simulink model "urineanalylsis"  (R2022a)
settings: Solver=VariableStepAuto  StartTime=0.0  StopTime=10.0  RelTol=1e-3
libraries: simulink x43, simulink_extras x1
settings Model: Creator=user  LastModifiedBy=hp

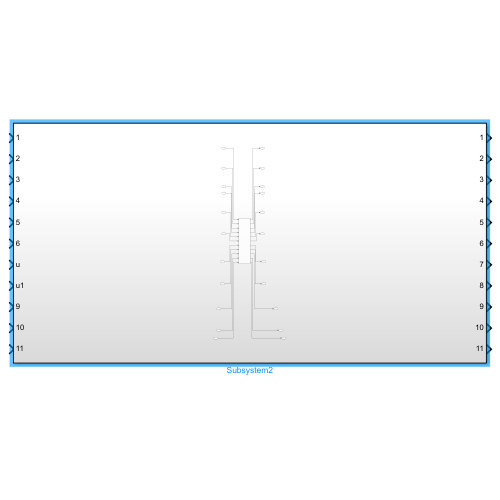
[thumbnail: Simulink's stored preview of the top-level diagram]
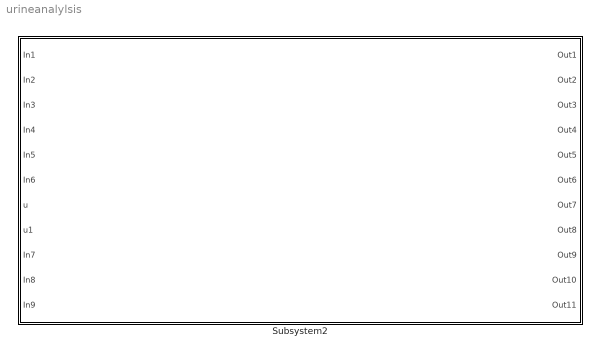
== system urineanalylsis ==
  Subsystem2 : Subsystem

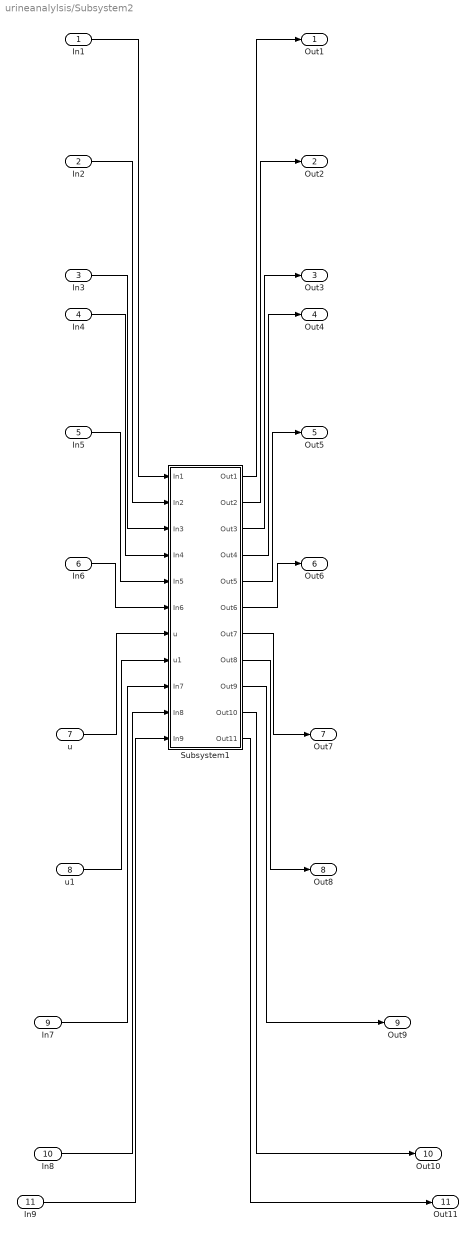
== system urineanalylsis/Subsystem2 ==
  In1 : Inport
  In2 : Inport  Port=2
  In3 : Inport  Port=3
  In4 : Inport  Port=4
  In5 : Inport  Port=5
  In6 : Inport  Port=6
  u : Inport  Port=7
  u1 : Inport  Port=8
  In7 : Inport  Port=9
  In8 : Inport  Port=10
  In9 : Inport  Port=11
  Subsystem1 : Subsystem
  Out1 : Outport
  Out2 : Outport  Port=2
  Out3 : Outport  Port=3
  Out4 : Outport  Port=4
  Out5 : Outport  Port=5
  Out6 : Outport  Port=6
  Out7 : Outport  Port=7
  Out8 : Outport  Port=8
  Out9 : Outport  Port=9
  Out10 : Outport  Port=10
  Out11 : Outport  Port=11
  wires:
  In1/1 -> Subsystem1/1(In1)
  In2/1 -> Subsystem1/2(In2)
  In3/1 -> Subsystem1/3(In3)
  In4/1 -> Subsystem1/4(In4)
  In5/1 -> Subsystem1/5(In5)
  In6/1 -> Subsystem1/6(In6)
  u/1 -> Subsystem1/7(u)
  u1/1 -> Subsystem1/8(u1)
  In7/1 -> Subsystem1/9(In7)
  In8/1 -> Subsystem1/10(In8)
  In9/1 -> Subsystem1/11(In9)
  Subsystem1/1(Out1) -> Out1/1
  Subsystem1/2(Out2) -> Out2/1
  Subsystem1/3(Out3) -> Out3/1
  Subsystem1/4(Out4) -> Out4/1
  Subsystem1/5(Out5) -> Out5/1
  Subsystem1/6(Out6) -> Out6/1
  Subsystem1/7(Out7) -> Out7/1
  Subsystem1/8(Out8) -> Out8/1
  Subsystem1/9(Out9) -> Out9/1
  Subsystem1/10(Out10) -> Out10/1
  Subsystem1/11(Out11) -> Out11/1

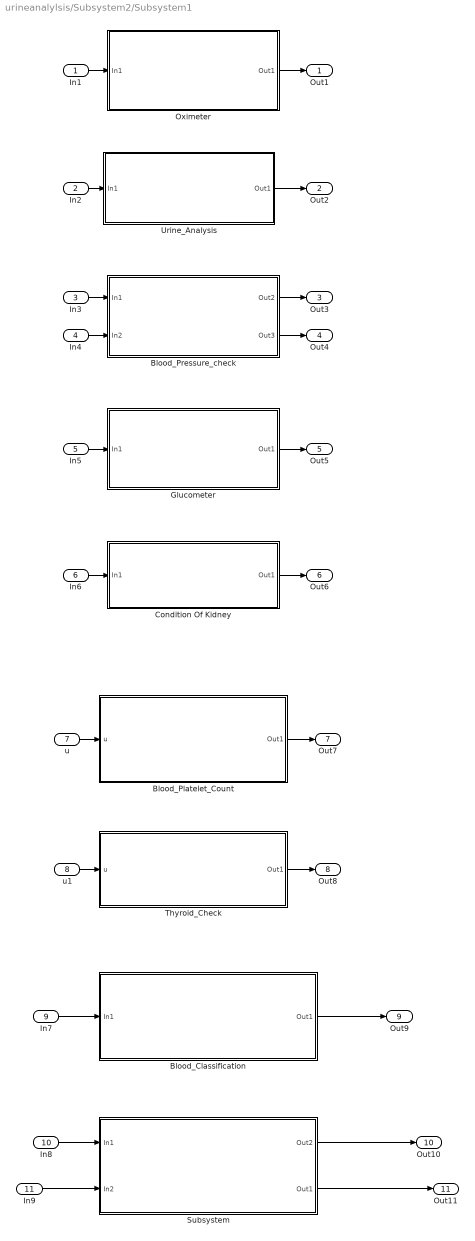
== system urineanalylsis/Subsystem2/Subsystem1 ==
  In1 : Inport
  In2 : Inport  Port=2
  In3 : Inport  Port=3
  In4 : Inport  Port=4
  In5 : Inport  Port=5
  In6 : Inport  Port=6
  u : Inport  Port=7
  u1 : Inport  Port=8
  In7 : Inport  Port=9
  In8 : Inport  Port=10
  In9 : Inport  Port=11
  Blood_Classification : Subsystem
  Blood_Platelet_Count : Subsystem
  Blood_Pressure_check : Subsystem
  Condition Of Kidney : Subsystem
  Glucometer : Subsystem
  Oximeter : Subsystem
  Subsystem : Subsystem
  Thyroid_Check : Subsystem
  Urine_Analysis : Subsystem
  Out1 : Outport
  Out2 : Outport  Port=2
  Out3 : Outport  Port=3
  Out4 : Outport  Port=4
  Out5 : Outport  Port=5
  Out6 : Outport  Port=6
  Out7 : Outport  Port=7
  Out8 : Outport  Port=8
  Out9 : Outport  Port=9
  Out10 : Outport  Port=10
  Out11 : Outport  Port=11
  wires:
  In6/1 -> Condition Of Kidney/1(In1)
  Subsystem/1(Out2) -> Out10/1
  In8/1 -> Subsystem/1(In1)
  In3/1 -> Blood_Pressure_check/1(In1)
  In4/1 -> Blood_Pressure_check/2(In2)
  In7/1 -> Blood_Classification/1(In1)
  u1/1 -> Thyroid_Check/1(u)
  In1/1 -> Oximeter/1(In1)
  u/1 -> Blood_Platelet_Count/1(u)
  Urine_Analysis/1(Out1) -> Out2/1
  Blood_Pressure_check/1(Out2) -> Out3/1
  Blood_Pressure_check/2(Out3) -> Out4/1
  Oximeter/1(Out1) -> Out1/1
  In2/1 -> Urine_Analysis/1(In1)
  Subsystem/2(Out1) -> Out11/1
  Thyroid_Check/1(Out1) -> Out8/1
  Condition Of Kidney/1(Out1) -> Out6/1
  Blood_Classification/1(Out1) -> Out9/1
  Blood_Platelet_Count/1(Out1) -> Out7/1
  In5/1 -> Glucometer/1(In1)
  Glucometer/1(Out1) -> Out5/1
  In9/1 -> Subsystem/2(In2)

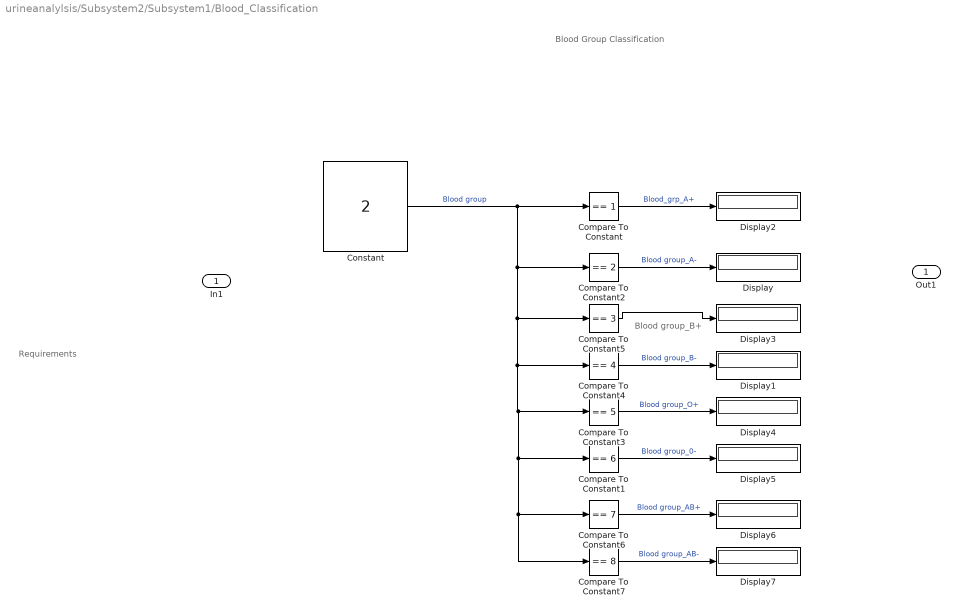
== system urineanalylsis/Subsystem2/Subsystem1/Blood_Classification ==
  note: Requirements
  note: Blood group_B+
  note: Blood Group Classification
  In1 : Inport
  Compare To Constant : simulink/Logic and Bit Operations/Compare To Constant  relop===  const=1  OutDataTypeStr=boolean
  Compare To Constant1 : simulink/Logic and Bit Operations/Compare To Constant  relop===  const=6  OutDataTypeStr=boolean
  Compare To Constant2 : simulink/Logic and Bit Operations/Compare To Constant  relop===  const=2  OutDataTypeStr=boolean
  Compare To Constant3 : simulink/Logic and Bit Operations/Compare To Constant  relop===  const=5  OutDataTypeStr=boolean
  Compare To Constant4 : simulink/Logic and Bit Operations/Compare To Constant  relop===  const=4  OutDataTypeStr=boolean
  Compare To Constant5 : simulink/Logic and Bit Operations/Compare To Constant  relop===  const=3  OutDataTypeStr=boolean
  Compare To Constant6 : simulink/Logic and Bit Operations/Compare To Constant  relop===  const=7  OutDataTypeStr=boolean
  Compare To Constant7 : simulink/Logic and Bit Operations/Compare To Constant  relop===  const=8  OutDataTypeStr=boolean
  Constant : Constant  Value=2
  Display{,1..7} (8 alike) : Display
  Out1 : Outport
  wires:
  Compare To Constant5/1 -> Display3/1
  Compare To Constant4/1 -> Display1/1  "Blood group_B-"
  Constant/1 -> Compare To Constant7/1, Compare To Constant6/1, Compare To Constant1/1, Compare To Constant3/1, Compare To Constant4/1, Compare To Constant5/1, Compare To Constant2/1, Compare To Constant/1  "Blood group"
  Compare To Constant6/1 -> Display6/1  "Blood group_AB+"
  Compare To Constant1/1 -> Display5/1  "Blood group_0-"
  Compare To Constant/1 -> Display2/1  "Blood_grp_A+"
  Compare To Constant2/1 -> Display/1  "Blood group_A-"
  Compare To Constant3/1 -> Display4/1  "Blood group_O+"
  Compare To Constant7/1 -> Display7/1  "Blood group_AB-"

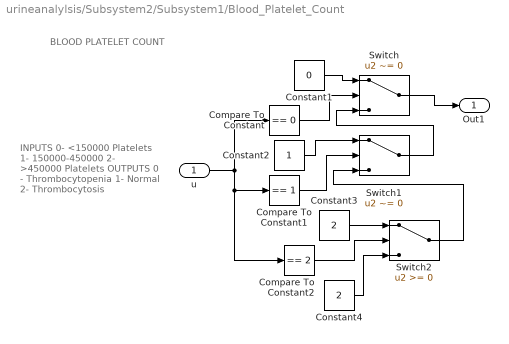
== system urineanalylsis/Subsystem2/Subsystem1/Blood_Platelet_Count ==
  note: BLOOD PLATELET COUNT
  note: INPUTS
      |
      | 0- <150000 Platelets
      | 1- 150000-450000
      | 2- >450000 Platelets
      |
      | OUTPUTS
      | 0 - Thrombocytopenia
      | 1-  Normal
      | 2-  Thrombocytosis
  u : Inport
  Compare To Constant : simulink/Logic and Bit Operations/Compare To Constant  relop===  const=0  OutDataTypeStr=boolean
  Compare To Constant1 : simulink/Logic and Bit Operations/Compare To Constant  relop===  const=1  OutDataTypeStr=boolean
  Compare To Constant2 : simulink/Logic and Bit Operations/Compare To Constant  relop===  const=2  OutDataTypeStr=boolean
  Constant1 : Constant  Value=0
  Constant2 : Constant
  Constant3 : Constant  Value=2
  Constant4 : Constant  Value=2
  Switch : Switch  Criteria=u2 ~= 0  SaturateOnIntegerOverflow=off  InputSameDT=off
  Switch1 : Switch  Criteria=u2 ~= 0  SaturateOnIntegerOverflow=off  InputSameDT=off
  Switch2 : Switch  SaturateOnIntegerOverflow=off  InputSameDT=off
  Out1 : Outport
  wires:
  Switch/1 -> Out1/1
  Constant2/1 -> Switch1/1
  Constant4/1 -> Switch2/3
  Compare To Constant/1 -> Switch/2
  Constant1/1 -> Switch/1
  Compare To Constant2/1 -> Switch2/2
  Compare To Constant1/1 -> Switch1/2
  Switch2/1 -> Switch1/3
  Constant3/1 -> Switch2/1
  Switch1/1 -> Switch/3
  u/1 -> Compare To Constant2/1, Compare To Constant1/1, Compare To Constant/1

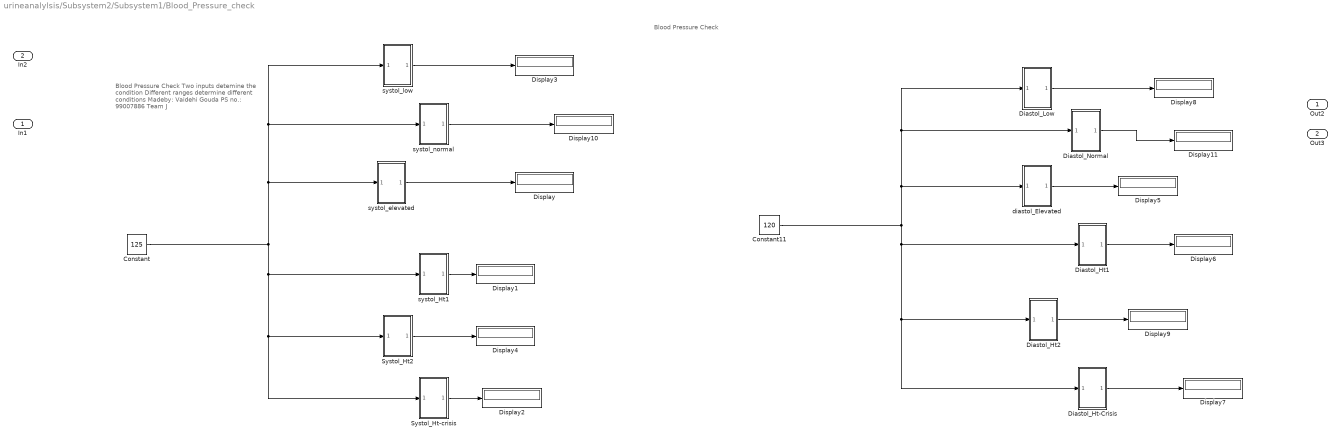
== system urineanalylsis/Subsystem2/Subsystem1/Blood_Pressure_check ==
  note: Blood Pressure Check
      |
      | Two inputs detemine the condition
      | Different ranges determine different conditions
      |
      | Madeby: Vaidehi Gouda
      | PS no.: 99007886
      | Team J
  note: Blood Pressure Check
  In1 : Inport
  In2 : Inport  Port=2
  Constant : Constant  Value=125
  Constant11 : Constant  Value=120
  Diastol_Ht-Crisis : Subsystem
  Diastol_Ht1 : Subsystem
  Diastol_Ht2 : Subsystem
  Diastol_Low : Subsystem
  Diastol_Normal : Subsystem
  Display{,1..11} (12 alike) : Display
  Systol_Ht-crisis : Subsystem
  Systol_Ht2 : Subsystem
  diastol_Elevated : Subsystem
  systol_Ht1 : Subsystem
  systol_elevated : Subsystem
  systol_low : Subsystem
  systol_normal : Subsystem
  Out2 : Outport
  Out3 : Outport  Port=2
  wires:
  Diastol_Ht2/1(Out1) -> Display9/1
  systol_Ht1/1(Out1) -> Display1/1
  Constant/1 -> Systol_Ht-crisis/1(In1), Systol_Ht2/1(In1), systol_Ht1/1(In1), systol_low/1(In1), systol_normal/1(In1), systol_elevated/1(In1)
  Diastol_Ht-Crisis/1(Out1) -> Display7/1
  Systol_Ht2/1(Out1) -> Display4/1
  Diastol_Normal/1(Out1) -> Display11/1
  systol_normal/1(Out1) -> Display10/1
  Constant11/1 -> Diastol_Ht-Crisis/1(In1), Diastol_Ht2/1(In1), Diastol_Ht1/1(In1), Diastol_Low/1(In1), Diastol_Normal/1(In1), diastol_Elevated/1(In1)
  diastol_Elevated/1(Out1) -> Display5/1
  Diastol_Low/1(Out1) -> Display8/1
  Diastol_Ht1/1(Out1) -> Display6/1
  systol_low/1(Out1) -> Display3/1
  Systol_Ht-crisis/1(Out1) -> Display2/1
  systol_elevated/1(Out1) -> Display/1

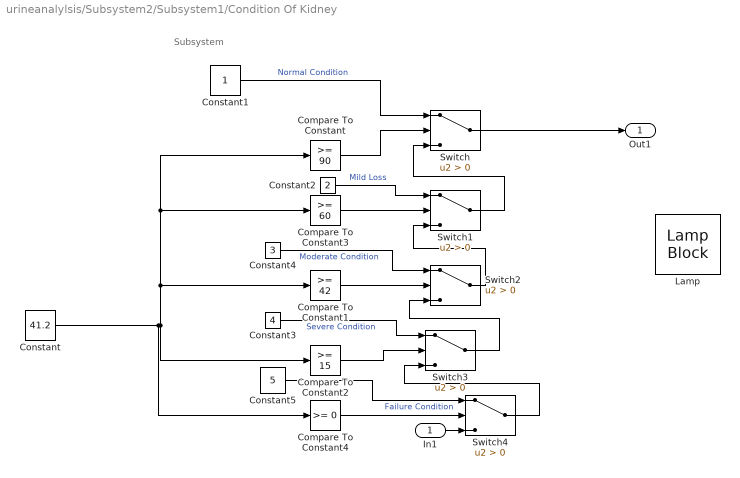
== system urineanalylsis/Subsystem2/Subsystem1/Condition Of Kidney ==
  note: Subsystem
  In1 : Inport
  Compare To Constant : simulink/Logic and Bit Operations/Compare To Constant  relop=>=  const=90  OutDataTypeStr=boolean
  Compare To Constant1 : simulink/Logic and Bit Operations/Compare To Constant  relop=>=  const=42  OutDataTypeStr=boolean
  Compare To Constant2 : simulink/Logic and Bit Operations/Compare To Constant  relop=>=  const=15  OutDataTypeStr=boolean
  Compare To Constant3 : simulink/Logic and Bit Operations/Compare To Constant  relop=>=  const=60  OutDataTypeStr=boolean
  Compare To Constant4 : simulink/Logic and Bit Operations/Compare To Constant  relop=>=  const=0  OutDataTypeStr=boolean
  Constant : Constant  Value=41.2
  Constant1 : Constant
  Constant2 : Constant  Value=2
  Constant3 : Constant  Value=4
  Constant4 : Constant  Value=3
  Constant5 : Constant  Value=5
  Lamp : LampBlock  LabelPosition=Hide
  Switch{,1..4} (5 alike) : Switch  Criteria=u2 > Threshold  SaturateOnIntegerOverflow=off  InputSameDT=off
  Out1 : Outport
  wires:
  Compare To Constant/1 -> Switch/2
  Constant1/1 -> Switch/1  "Normal Condition"
  Compare To Constant4/1 -> Switch4/2
  Switch2/1 -> Switch1/3
  Constant/1 -> Compare To Constant3/1, Compare To Constant/1, Compare To Constant1/1, Compare To Constant2/1, Compare To Constant4/1
  Switch4/1 -> Switch3/3
  Switch1/1 -> Switch/3
  Compare To Constant1/1 -> Switch2/2
  Switch3/1 -> Switch2/3
  Constant3/1 -> Switch3/1  "Severe Condition"
  Constant4/1 -> Switch2/1  "Moderate Condition"
  Compare To Constant2/1 -> Switch3/2
  Compare To Constant3/1 -> Switch1/2
  Constant2/1 -> Switch1/1  "Mild Loss"
  Constant5/1 -> Switch4/1  "Failure Condition"
  In1/1 -> Switch4/3
  Switch/1 -> Out1/1

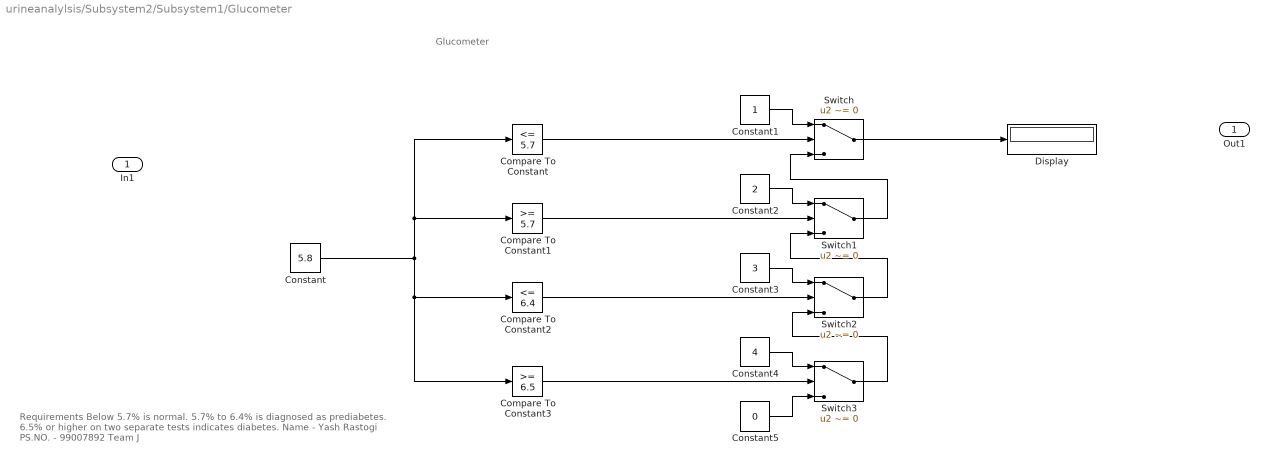
== system urineanalylsis/Subsystem2/Subsystem1/Glucometer ==
  note: Glucometer
  note: Requirements
      |
      | Below 5.7% is normal.
      | 5.7% to 6.4% is diagnosed as prediabetes.
      | 6.5% or higher on two separate tests indicates diabetes.
      | Name - Yash Rastogi
      | PS.NO. - 99007892
      | Team J
  In1 : Inport
  Compare To Constant : simulink/Logic and Bit Operations/Compare To Constant  relop=<=  const=5.7  OutDataTypeStr=boolean
  Compare To Constant1 : simulink/Logic and Bit Operations/Compare To Constant  relop=>=  const=5.7  OutDataTypeStr=boolean
  Compare To Constant2 : simulink/Logic and Bit Operations/Compare To Constant  relop=<=  const=6.4  OutDataTypeStr=boolean
  Compare To Constant3 : simulink/Logic and Bit Operations/Compare To Constant  relop=>=  const=6.5  OutDataTypeStr=boolean
  Constant : Constant  Value=5.8
  Constant1 : Constant
  Constant2 : Constant  Value=2
  Constant3 : Constant  Value=3
  Constant4 : Constant  Value=4
  Constant5 : Constant  Value=0
  Display : Display
  Switch{,1..3} (4 alike) : Switch  Criteria=u2 ~= 0  SaturateOnIntegerOverflow=off  InputSameDT=off
  Out1 : Outport
  wires:
  Compare To Constant1/1 -> Switch1/2
  Compare To Constant3/1 -> Switch3/2
  Compare To Constant/1 -> Switch/2
  Switch1/1 -> Switch/3
  Constant/1 -> Compare To Constant3/1, Compare To Constant2/1, Compare To Constant1/1, Compare To Constant/1
  Constant4/1 -> Switch3/1
  Switch2/1 -> Switch1/3
  Switch3/1 -> Switch2/3
  Constant5/1 -> Switch3/3
  Compare To Constant2/1 -> Switch2/2
  Constant1/1 -> Switch/1
  Constant2/1 -> Switch1/1
  Switch/1 -> Display/1
  Constant3/1 -> Switch2/1

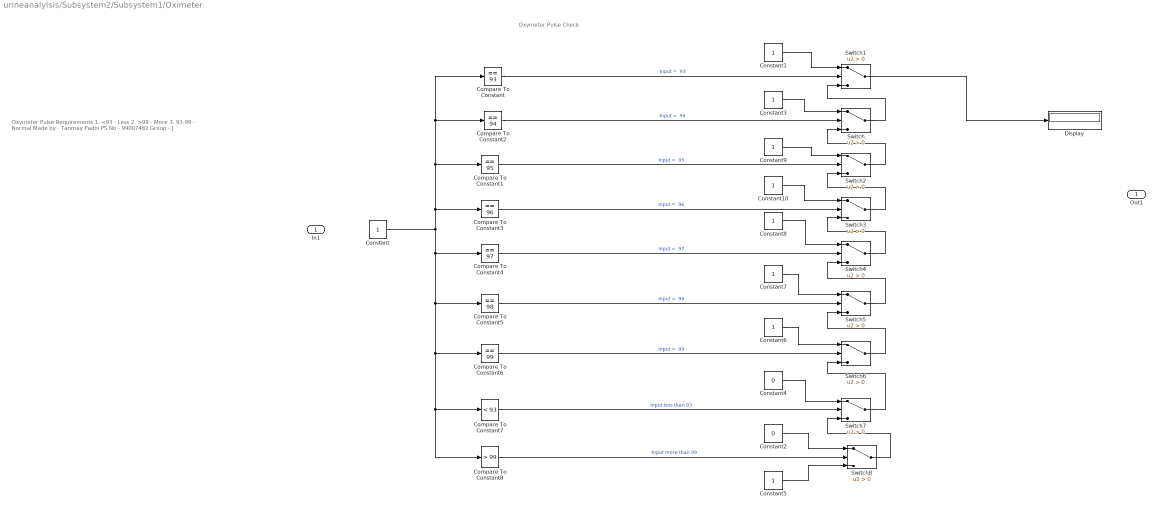
== system urineanalylsis/Subsystem2/Subsystem1/Oximeter ==
  note: Oxymeter Pulse
      |
      | Requirements
      | 1. <93 - Less
      | 2. >99 - More
      | 3. 93-99 - Normal
      |
      | Made by - Tanmay Padhi
      | PS No - 99007482
      | Group - J
  note: Oxymeter Pulse Check
  In1 : Inport
  Compare To Constant : simulink/Logic and Bit Operations/Compare To Constant  relop===  const=93  OutDataTypeStr=boolean
  Compare To Constant1 : simulink/Logic and Bit Operations/Compare To Constant  relop===  const=95  OutDataTypeStr=boolean
  Compare To Constant2 : simulink/Logic and Bit Operations/Compare To Constant  relop===  const=94  OutDataTypeStr=boolean
  Compare To Constant3 : simulink/Logic and Bit Operations/Compare To Constant  relop===  const=96  OutDataTypeStr=boolean
  Compare To Constant4 : simulink/Logic and Bit Operations/Compare To Constant  relop===  const=97  OutDataTypeStr=boolean
  Compare To Constant5 : simulink/Logic and Bit Operations/Compare To Constant  relop===  const=98  OutDataTypeStr=boolean
  Compare To Constant6 : simulink/Logic and Bit Operations/Compare To Constant  relop===  const=99  OutDataTypeStr=boolean
  Compare To Constant7 : simulink/Logic and Bit Operations/Compare To Constant  relop=<  const=93  OutDataTypeStr=boolean
  Compare To Constant8 : simulink/Logic and Bit Operations/Compare To Constant  relop=>  const=99  OutDataTypeStr=boolean
  Constant{,1,3,5..10} (9 alike) : Constant
  Constant2 : Constant  Value=0
  Constant4 : Constant  Value=0
  Display : Display
  Switch{,1..8} (9 alike) : Switch  Criteria=u2 > Threshold  SaturateOnIntegerOverflow=off  InputSameDT=off
  Out1 : Outport
  wires:
  Switch7/1 -> Switch6/3
  Compare To Constant4/1 -> Switch4/2  "Input =  97"
  Constant1/1 -> Switch1/1
  Compare To Constant7/1 -> Switch7/2  "Input less than 93"
  Switch6/1 -> Switch5/3
  Constant/1 -> Compare To Constant4/1, Compare To Constant5/1, Compare To Constant8/1, Compare To Constant7/1, Compare To Constant6/1, Compare To Constant2/1, Compare To Constant/1, Compare To Constant1/1, Compare To Constant3/1
  Compare To Constant5/1 -> Switch5/2  "Input =  98"
  Switch4/1 -> Switch3/3
  Constant9/1 -> Switch2/1
  Compare To Constant/1 -> Switch1/2  "Input =  93"
  Compare To Constant1/1 -> Switch2/2  "Input =  95"
  Constant5/1 -> Switch8/3
  Constant3/1 -> Switch/1
  Switch3/1 -> Switch2/3
  Switch2/1 -> Switch/3
  Constant8/1 -> Switch4/1
  Compare To Constant3/1 -> Switch3/2  "Input =  96"
  Switch/1 -> Switch1/3
  Compare To Constant8/1 -> Switch8/2  "Input more than 99"
  Constant6/1 -> Switch6/1
  Constant4/1 -> Switch7/1
  Switch8/1 -> Switch7/3
  Constant7/1 -> Switch5/1
  Compare To Constant6/1 -> Switch6/2  "Input =  99"
  Switch5/1 -> Switch4/3
  Compare To Constant2/1 -> Switch/2  "Input =  94"
  Constant2/1 -> Switch8/1
  Constant10/1 -> Switch3/1
  Switch1/1 -> Display/1

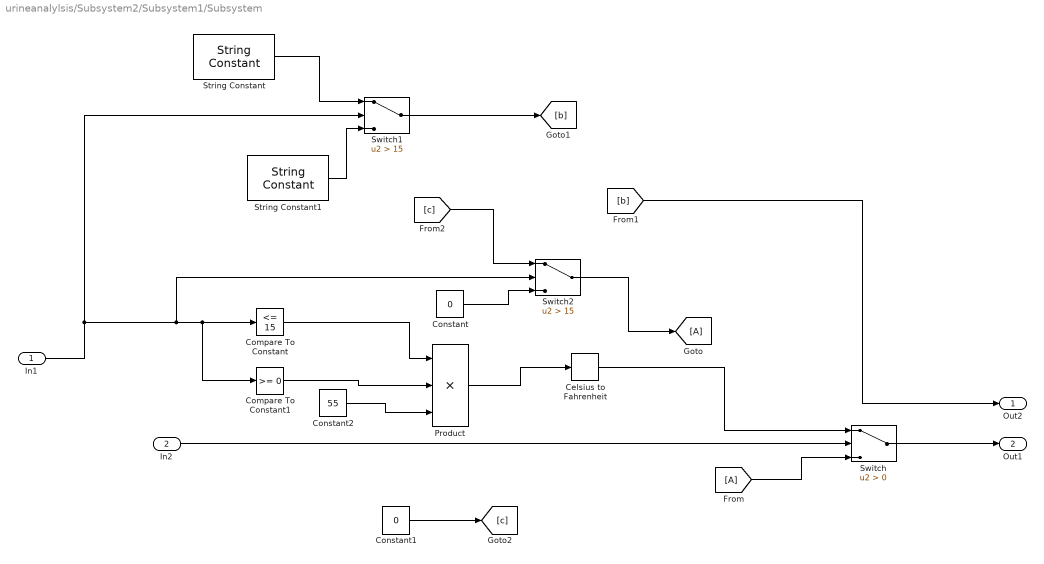
== system urineanalylsis/Subsystem2/Subsystem1/Subsystem ==
  In1 : Inport
  In2 : Inport  Port=2
  Celsius to Fahrenheit : simulink_extras/Transformations/Celsius to Fahrenheit
      settings: SourceProductBaseCode=SL
  Compare To Constant : simulink/Logic and Bit Operations/Compare To Constant  relop=<=  const=15  OutDataTypeStr=boolean
  Compare To Constant1 : simulink/Logic and Bit Operations/Compare To Constant  relop=>=  const=0  OutDataTypeStr=boolean
  Constant : Constant  Value=0
  Constant1 : Constant  Value=0
  Constant2 : Constant  Value=55
  From : From
  Goto : Goto
  Product : Product  Inputs=3
  String Constant : StringConstant  String="\"invalid\""
  String Constant1 : StringConstant  String="\"working\""
  Switch : Switch  Criteria=u2 > Threshold  SaturateOnIntegerOverflow=off  InputSameDT=off
  Switch1 : Switch  Criteria=u2 > Threshold  Threshold=15  SaturateOnIntegerOverflow=off  InputSameDT=off
  Switch2 : Switch  Criteria=u2 > Threshold  Threshold=15  SaturateOnIntegerOverflow=off  InputSameDT=off
  Out2 : Outport
  Out1 : Outport  Port=2
  wires:
  Product/1 -> Celsius to Fahrenheit/1
  In2/1 -> Switch/2
  Switch/1 -> Out1/1
  Celsius to Fahrenheit/1 -> Switch/1
  From/1 -> Switch/3
  Constant2/1 -> Product/3
  Compare To Constant/1 -> Product/1
  Compare To Constant1/1 -> Product/2
  String Constant/1 -> Switch1/1
  Switch1/1 -> [b]
  [b] -> Out2/1
  String Constant1/1 -> Switch1/3
  In1/1 -> Switch2/2, Compare To Constant1/1, Compare To Constant/1, Switch1/2
  Switch2/1 -> Goto/1
  Constant/1 -> Switch2/3
  [c] -> Switch2/1
  Constant1/1 -> [c]

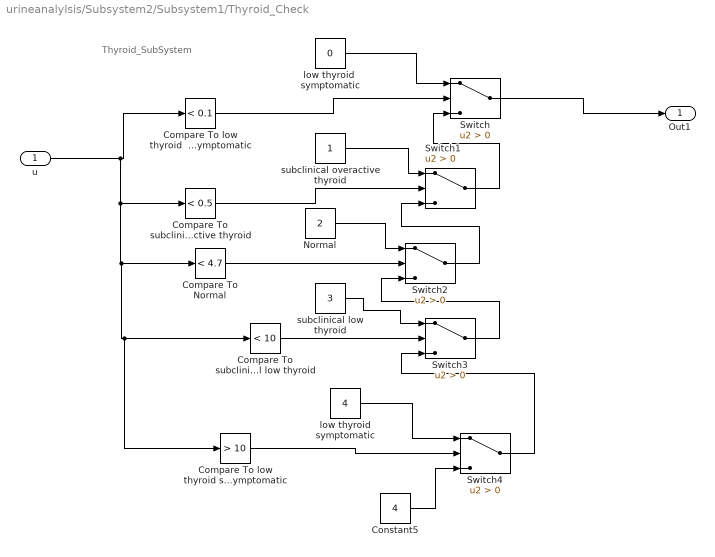
== system urineanalylsis/Subsystem2/Subsystem1/Thyroid_Check ==
  note: Thyroid_SubSystem
  u : Inport
  Compare To Normal : simulink/Logic and Bit Operations/Compare To Constant  relop=<  const=4.7  OutDataTypeStr=boolean
  Compare To low thyroid  symptomatic : simulink/Logic and Bit Operations/Compare To Constant  relop=<  const=0.1  OutDataTypeStr=boolean
  Compare To low thyroid symptomatic : simulink/Logic and Bit Operations/Compare To Constant  relop=>  const=10  OutDataTypeStr=boolean
  "Compare To subclinical low thyroid " : simulink/Logic and Bit Operations/Compare To Constant  relop=<  const=10  OutDataTypeStr=boolean
  Compare To subclinical overactive thyroid : simulink/Logic and Bit Operations/Compare To Constant  relop=<  const=0.5  OutDataTypeStr=boolean
  Constant5 : Constant  Value=4
  Normal : Constant  Value=2
  Switch{,1..4} (5 alike) : Switch  Criteria=u2 > Threshold  SaturateOnIntegerOverflow=off  InputSameDT=off
  low thyroid  symptomatic : Constant  Value=0
  low thyroid symptomatic : Constant  Value=4
  subclinical low thyroid : Constant  Value=3
  subclinical overactive thyroid : Constant
  Out1 : Outport
  wires:
  Compare To low thyroid  symptomatic/1 -> Switch/2
  Switch/1 -> Out1/1
  low thyroid  symptomatic/1 -> Switch/1
  Constant5/1 -> Switch4/3
  Switch3/1 -> Switch2/3
  u/1 -> Compare To low thyroid symptomatic/1, "Compare To subclinical low thyroid "/1, Compare To Normal/1, Compare To subclinical overactive thyroid/1, Compare To low thyroid  symptomatic/1
  "Compare To subclinical low thyroid "/1 -> Switch3/2
  Switch1/1 -> Switch/3
  Compare To low thyroid symptomatic/1 -> Switch4/2
  Switch4/1 -> Switch3/3
  Normal/1 -> Switch2/1
  Switch2/1 -> Switch1/3
  Compare To subclinical overactive thyroid/1 -> Switch1/2
  low thyroid symptomatic/1 -> Switch4/1
  subclinical low thyroid/1 -> Switch3/1
  Compare To Normal/1 -> Switch2/2
  subclinical overactive thyroid/1 -> Switch1/1

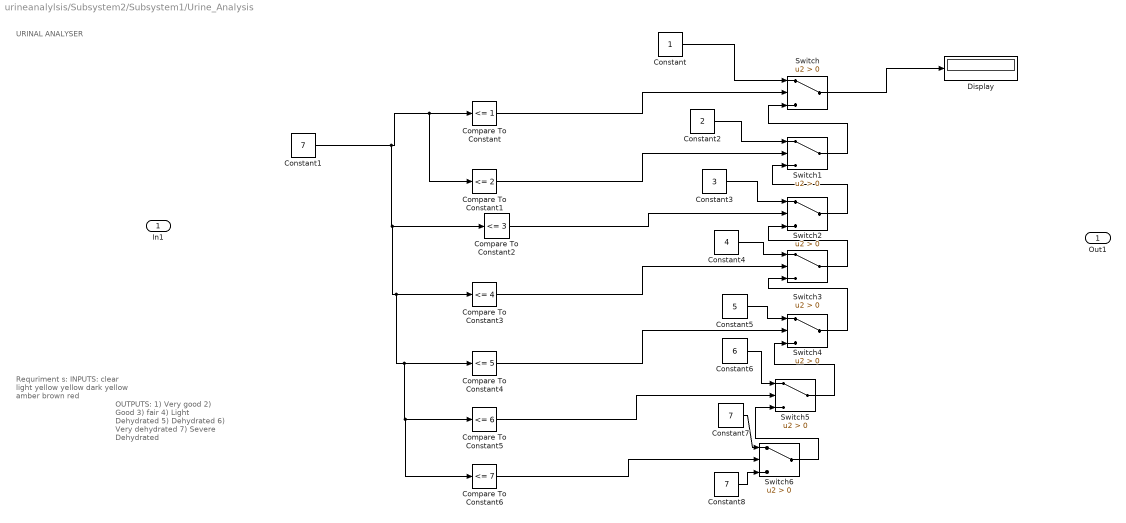
== system urineanalylsis/Subsystem2/Subsystem1/Urine_Analysis ==
  note: OUTPUTS:
      |  1) Very good
      | 2) Good
      | 3) fair
      | 4) Light Dehydrated
      | 5) Dehydrated
      | 6) Very dehydrated
      | 7) Severe Dehydrated
  note: Requriment s:
      | INPUTS:
      | clear
      | light yellow
      | yellow
      | dark yellow
      | amber
      | brown
      | red
  note: URINAL ANALYSER
  In1 : Inport
  Compare To Constant : simulink/Logic and Bit Operations/Compare To Constant  relop=<=  const=1  OutDataTypeStr=boolean
  Compare To Constant1 : simulink/Logic and Bit Operations/Compare To Constant  relop=<=  const=2  OutDataTypeStr=boolean
  Compare To Constant2 : simulink/Logic and Bit Operations/Compare To Constant  relop=<=  const=3  OutDataTypeStr=boolean
  Compare To Constant3 : simulink/Logic and Bit Operations/Compare To Constant  relop=<=  const=4  OutDataTypeStr=boolean
  Compare To Constant4 : simulink/Logic and Bit Operations/Compare To Constant  relop=<=  const=5  OutDataTypeStr=boolean
  Compare To Constant5 : simulink/Logic and Bit Operations/Compare To Constant  relop=<=  const=6  OutDataTypeStr=boolean
  Compare To Constant6 : simulink/Logic and Bit Operations/Compare To Constant  relop=<=  const=7  OutDataTypeStr=boolean
  Constant : Constant
  Constant1 : Constant  Value=7
  Constant2 : Constant  Value=2
  Constant3 : Constant  Value=3
  Constant4 : Constant  Value=4
  Constant5 : Constant  Value=5
  Constant6 : Constant  Value=6
  Constant7 : Constant  Value=7
  Constant8 : Constant  Value=7
  Display : Display
  Switch{,1..6} (7 alike) : Switch  Criteria=u2 > Threshold  SaturateOnIntegerOverflow=off  InputSameDT=off
  Out1 : Outport
  wires:
  Constant/1 -> Switch/1
  Constant1/1 -> Compare To Constant6/1, Compare To Constant5/1, Compare To Constant4/1, Compare To Constant3/1, Compare To Constant2/1, Compare To Constant1/1, Compare To Constant/1
  Constant2/1 -> Switch1/1
  Compare To Constant5/1 -> Switch5/2
  Compare To Constant2/1 -> Switch2/2
  Compare To Constant/1 -> Switch/2
  Compare To Constant1/1 -> Switch1/2
  Constant5/1 -> Switch4/1
  Constant6/1 -> Switch5/1
  Switch6/1 -> Switch5/3
  Switch2/1 -> Switch1/3
  Switch4/1 -> Switch3/3
  Compare To Constant4/1 -> Switch4/2
  Switch1/1 -> Switch/3
  Constant4/1 -> Switch3/1
  Switch3/1 -> Switch2/3
  Compare To Constant3/1 -> Switch3/2
  Switch/1 -> Display/1
  Compare To Constant6/1 -> Switch6/2
  Constant3/1 -> Switch2/1
  Switch5/1 -> Switch4/3
  Constant8/1 -> Switch6/3
  Constant7/1 -> Switch6/1

== system urineanalylsis/Subsystem2/Subsystem1/Blood_Pressure_check/Diastol_Ht-Crisis ==
  In1 : Inport
  Constant18 : Constant
  Constant21 : Constant
  If Action Subsystem16 : Subsystem  TreatAsAtomicUnit=on
  If Action Subsystem19 : Subsystem  TreatAsAtomicUnit=on
  If16 : If  IfExpression=u1 >=120  ShowElse=off
  If17 : If  IfExpression=u1 <=170  ShowElse=off
  Logical Operator7 : Logic  AllPortsSameDT=off  OutDataTypeStr=boolean
  Out1 : Outport
  wires:
  If Action Subsystem19/1(Out1) -> Logical Operator7/2
  Constant18/1 -> If Action Subsystem16/1(In1)
  In1/1 -> If17/1, If16/1
  If Action Subsystem16/1(Out1) -> Logical Operator7/1
  If16/1 -> If Action Subsystem16/Action
  Constant21/1 -> If Action Subsystem19/1(In1)
  If17/1 -> If Action Subsystem19/Action
  Logical Operator7/1 -> Out1/1

== system urineanalylsis/Subsystem2/Subsystem1/Blood_Pressure_check/Diastol_Ht1 ==
  In1 : Inport
  Constant15 : Constant
  Constant16 : Constant
  If Action Subsystem12 : Subsystem  TreatAsAtomicUnit=on
  If Action Subsystem13 : Subsystem  TreatAsAtomicUnit=on
  If12 : If  IfExpression=u1 >=80  ShowElse=off
  If13 : If  IfExpression=u1 <=89  ShowElse=off
  Logical Operator6 : Logic  AllPortsSameDT=off  OutDataTypeStr=boolean
  Out1 : Outport
  wires:
  If12/1 -> If Action Subsystem12/Action
  If Action Subsystem12/1(Out1) -> Logical Operator6/1
  Constant16/1 -> If Action Subsystem13/1(In1)
  If Action Subsystem13/1(Out1) -> Logical Operator6/2
  Constant15/1 -> If Action Subsystem12/1(In1)
  In1/1 -> If13/1, If12/1
  If13/1 -> If Action Subsystem13/Action
  Logical Operator6/1 -> Out1/1

== system urineanalylsis/Subsystem2/Subsystem1/Blood_Pressure_check/Diastol_Ht2 ==
  In1 : Inport
  Constant17 : Constant
  Constant19 : Constant
  If Action Subsystem14 : Subsystem  TreatAsAtomicUnit=on
  If Action Subsystem15 : Subsystem  TreatAsAtomicUnit=on
  If14 : If  IfExpression=u1 >=90  ShowElse=off
  If15 : If  IfExpression=u1 <=99  ShowElse=off
  Logical Operator9 : Logic  AllPortsSameDT=off  OutDataTypeStr=boolean
  Out1 : Outport
  wires:
  If14/1 -> If Action Subsystem14/Action
  In1/1 -> If15/1, If14/1
  Constant17/1 -> If Action Subsystem14/1(In1)
  If Action Subsystem15/1(Out1) -> Logical Operator9/2
  If15/1 -> If Action Subsystem15/Action
  Constant19/1 -> If Action Subsystem15/1(In1)
  If Action Subsystem14/1(Out1) -> Logical Operator9/1
  Logical Operator9/1 -> Out1/1

== system urineanalylsis/Subsystem2/Subsystem1/Blood_Pressure_check/Diastol_Low ==
  In1 : Inport
  Constant13 : Constant
  Constant20 : Constant
  If Action Subsystem17 : Subsystem  TreatAsAtomicUnit=on
  If Action Subsystem18 : Subsystem  TreatAsAtomicUnit=on
  If18 : If  IfExpression=u1 >=60  ShowElse=off
  If19 : If  IfExpression=u1 <=74  ShowElse=off
  Logical Operator8 : Logic  AllPortsSameDT=off  OutDataTypeStr=boolean
  Out1 : Outport
  wires:
  Constant20/1 -> If Action Subsystem17/1(In1)
  If18/1 -> If Action Subsystem17/Action
  Constant13/1 -> If Action Subsystem18/1(In1)
  If Action Subsystem18/1(Out1) -> Logical Operator8/2
  If Action Subsystem17/1(Out1) -> Logical Operator8/1
  In1/1 -> If18/1, If19/1
  If19/1 -> If Action Subsystem18/Action
  Logical Operator8/1 -> Out1/1

== system urineanalylsis/Subsystem2/Subsystem1/Blood_Pressure_check/Diastol_Normal ==
  In1 : Inport
  Constant23 : Constant
  If Action Subsystem21 : Subsystem  TreatAsAtomicUnit=on
  If21 : If  IfExpression=u1 == 80  ShowElse=off
  Out1 : Outport
  wires:
  Constant23/1 -> If Action Subsystem21/1(In1)
  If21/1 -> If Action Subsystem21/Action
  In1/1 -> If21/1
  If Action Subsystem21/1(Out1) -> Out1/1

== system urineanalylsis/Subsystem2/Subsystem1/Blood_Pressure_check/Systol_Ht-crisis ==
  In1 : Inport
  Constant6 : Constant
  Constant7 : Constant
  If Action Subsystem6 : Subsystem  TreatAsAtomicUnit=on
  If Action Subsystem7 : Subsystem  TreatAsAtomicUnit=on
  If6 : If  IfExpression=u1 >=180  ShowElse=off
  If7 : If  IfExpression=u1 <=260  ShowElse=off
  Logical Operator2 : Logic  AllPortsSameDT=off  OutDataTypeStr=boolean
  Out1 : Outport
  wires:
  Constant6/1 -> If Action Subsystem6/1(In1)
  In1/1 -> If6/1, If7/1
  Logical Operator2/1 -> Out1/1
  Constant7/1 -> If Action Subsystem7/1(In1)
  If7/1 -> If Action Subsystem7/Action
  If Action Subsystem6/1(Out1) -> Logical Operator2/1
  If6/1 -> If Action Subsystem6/Action
  If Action Subsystem7/1(Out1) -> Logical Operator2/2

== system urineanalylsis/Subsystem2/Subsystem1/Blood_Pressure_check/Systol_Ht2 ==
  In1 : Inport
  Constant5 : Constant
  Constant8 : Constant
  If Action Subsystem4 : Subsystem  TreatAsAtomicUnit=on
  If Action Subsystem5 : Subsystem  TreatAsAtomicUnit=on
  If4 : If  IfExpression=u1 >=140  ShowElse=off
  If5 : If  IfExpression=u1 <=159  ShowElse=off
  Logical Operator4 : Logic  AllPortsSameDT=off  OutDataTypeStr=boolean
  Out1 : Outport
  wires:
  Logical Operator4/1 -> Out1/1
  If5/1 -> If Action Subsystem5/Action
  If Action Subsystem4/1(Out1) -> Logical Operator4/1
  Constant8/1 -> If Action Subsystem5/1(In1)
  In1/1 -> If5/1, If4/1
  If Action Subsystem5/1(Out1) -> Logical Operator4/2
  Constant5/1 -> If Action Subsystem4/1(In1)
  If4/1 -> If Action Subsystem4/Action

== system urineanalylsis/Subsystem2/Subsystem1/Blood_Pressure_check/diastol_Elevated ==
  In1 : Inport
  Constant12 : Constant
  Constant14 : Constant
  If Action Subsystem10 : Subsystem  TreatAsAtomicUnit=on
  If Action Subsystem11 : Subsystem  TreatAsAtomicUnit=on
  If10 : If  IfExpression=u1 > 75  ShowElse=off
  If11 : If  IfExpression=u1 <=80  ShowElse=off
  Logical Operator5 : Logic  AllPortsSameDT=off  OutDataTypeStr=boolean
  Out1 : Outport
  wires:
  Constant12/1 -> If Action Subsystem10/1(In1)
  Logical Operator5/1 -> Out1/1
  If Action Subsystem11/1(Out1) -> Logical Operator5/2
  In1/1 -> If11/1, If10/1
  If Action Subsystem10/1(Out1) -> Logical Operator5/1
  Constant14/1 -> If Action Subsystem11/1(In1)
  If11/1 -> If Action Subsystem11/Action
  If10/1 -> If Action Subsystem10/Action

== system urineanalylsis/Subsystem2/Subsystem1/Blood_Pressure_check/systol_Ht1 ==
  In1 : Inport
  Constant3 : Constant
  Constant4 : Constant
  If Action Subsystem2 : Subsystem  TreatAsAtomicUnit=on
  If Action Subsystem3 : Subsystem  TreatAsAtomicUnit=on
  If2 : If  IfExpression=u1 >=130  ShowElse=off
  If3 : If  IfExpression=u1 <=139  ShowElse=off
  Logical Operator1 : Logic  AllPortsSameDT=off  OutDataTypeStr=boolean
  Out1 : Outport
  wires:
  If2/1 -> If Action Subsystem2/Action
  Logical Operator1/1 -> Out1/1
  Constant3/1 -> If Action Subsystem2/1(In1)
  If Action Subsystem2/1(Out1) -> Logical Operator1/1
  If3/1 -> If Action Subsystem3/Action
  Constant4/1 -> If Action Subsystem3/1(In1)
  In1/1 -> If3/1, If2/1
  If Action Subsystem3/1(Out1) -> Logical Operator1/2

== system urineanalylsis/Subsystem2/Subsystem1/Blood_Pressure_check/systol_elevated ==
  In1 : Inport
  Constant1 : Constant
  Constant2 : Constant
  If : If  IfExpression=u1 > 120  ShowElse=off
  If Action Subsystem : Subsystem  TreatAsAtomicUnit=on
  If Action Subsystem1 : Subsystem  TreatAsAtomicUnit=on
  If1 : If  IfExpression=u1 <=129  ShowElse=off
  Logical Operator : Logic  AllPortsSameDT=off  OutDataTypeStr=boolean
  Out1 : Outport
  wires:
  If Action Subsystem/1(Out1) -> Logical Operator/1
  Constant2/1 -> If Action Subsystem1/1(In1)
  If1/1 -> If Action Subsystem1/Action
  Constant1/1 -> If Action Subsystem/1(In1)
  In1/1 -> If1/1, If/1
  If/1 -> If Action Subsystem/Action
  If Action Subsystem1/1(Out1) -> Logical Operator/2
  Logical Operator/1 -> Out1/1

== system urineanalylsis/Subsystem2/Subsystem1/Blood_Pressure_check/systol_low ==
  In1 : Inport
  Constant10 : Constant
  Constant9 : Constant
  If Action Subsystem8 : Subsystem  TreatAsAtomicUnit=on
  If Action Subsystem9 : Subsystem  TreatAsAtomicUnit=on
  If8 : If  IfExpression=u1 >=90  ShowElse=off
  If9 : If  IfExpression=u1 <=100  ShowElse=off
  Logical Operator3 : Logic  AllPortsSameDT=off  OutDataTypeStr=boolean
  Out1 : Outport
  wires:
  Constant10/1 -> If Action Subsystem9/1(In1)
  In1/1 -> If9/1, If8/1
  If Action Subsystem8/1(Out1) -> Logical Operator3/1
  If8/1 -> If Action Subsystem8/Action
  Constant9/1 -> If Action Subsystem8/1(In1)
  If9/1 -> If Action Subsystem9/Action
  If Action Subsystem9/1(Out1) -> Logical Operator3/2
  Logical Operator3/1 -> Out1/1

== system urineanalylsis/Subsystem2/Subsystem1/Blood_Pressure_check/systol_normal ==
  In1 : Inport
  Constant22 : Constant
  If Action Subsystem20 : Subsystem  TreatAsAtomicUnit=on
  If20 : If  IfExpression=u1 == 120  ShowElse=off
  Out1 : Outport
  wires:
  If20/1 -> If Action Subsystem20/Action
  If Action Subsystem20/1(Out1) -> Out1/1
  Constant22/1 -> If Action Subsystem20/1(In1)
  In1/1 -> If20/1

== system urineanalylsis/Subsystem2/Subsystem1/Blood_Pressure_check/Diastol_Ht-Crisis/If Action Subsystem16 ==
  In1 : Inport
  Action Port : ActionPort
  Out1 : Outport
  wires:
  In1/1 -> Out1/1

== system urineanalylsis/Subsystem2/Subsystem1/Blood_Pressure_check/Diastol_Ht-Crisis/If Action Subsystem19 ==
  In1 : Inport
  Action Port : ActionPort
  Out1 : Outport
  wires:
  In1/1 -> Out1/1

== system urineanalylsis/Subsystem2/Subsystem1/Blood_Pressure_check/Diastol_Ht1/If Action Subsystem12 ==
  In1 : Inport
  Action Port : ActionPort
  Out1 : Outport
  wires:
  In1/1 -> Out1/1

== system urineanalylsis/Subsystem2/Subsystem1/Blood_Pressure_check/Diastol_Ht1/If Action Subsystem13 ==
  In1 : Inport
  Action Port : ActionPort
  Out1 : Outport
  wires:
  In1/1 -> Out1/1

== system urineanalylsis/Subsystem2/Subsystem1/Blood_Pressure_check/Diastol_Ht2/If Action Subsystem14 ==
  In1 : Inport
  Action Port : ActionPort
  Out1 : Outport
  wires:
  In1/1 -> Out1/1

== system urineanalylsis/Subsystem2/Subsystem1/Blood_Pressure_check/Diastol_Ht2/If Action Subsystem15 ==
  In1 : Inport
  Action Port : ActionPort
  Out1 : Outport
  wires:
  In1/1 -> Out1/1

== system urineanalylsis/Subsystem2/Subsystem1/Blood_Pressure_check/Diastol_Low/If Action Subsystem17 ==
  In1 : Inport
  Action Port : ActionPort
  Out1 : Outport
  wires:
  In1/1 -> Out1/1

== system urineanalylsis/Subsystem2/Subsystem1/Blood_Pressure_check/Diastol_Low/If Action Subsystem18 ==
  In1 : Inport
  Action Port : ActionPort
  Out1 : Outport
  wires:
  In1/1 -> Out1/1

== system urineanalylsis/Subsystem2/Subsystem1/Blood_Pressure_check/Diastol_Normal/If Action Subsystem21 ==
  In1 : Inport
  Action Port : ActionPort
  Out1 : Outport
  wires:
  In1/1 -> Out1/1

== system urineanalylsis/Subsystem2/Subsystem1/Blood_Pressure_check/Systol_Ht-crisis/If Action Subsystem6 ==
  In1 : Inport
  Action Port : ActionPort
  Out1 : Outport
  wires:
  In1/1 -> Out1/1

== system urineanalylsis/Subsystem2/Subsystem1/Blood_Pressure_check/Systol_Ht-crisis/If Action Subsystem7 ==
  In1 : Inport
  Action Port : ActionPort
  Out1 : Outport
  wires:
  In1/1 -> Out1/1

== system urineanalylsis/Subsystem2/Subsystem1/Blood_Pressure_check/Systol_Ht2/If Action Subsystem4 ==
  In1 : Inport
  Action Port : ActionPort
  Out1 : Outport
  wires:
  In1/1 -> Out1/1

== system urineanalylsis/Subsystem2/Subsystem1/Blood_Pressure_check/Systol_Ht2/If Action Subsystem5 ==
  In1 : Inport
  Action Port : ActionPort
  Out1 : Outport
  wires:
  In1/1 -> Out1/1

== system urineanalylsis/Subsystem2/Subsystem1/Blood_Pressure_check/diastol_Elevated/If Action Subsystem10 ==
  In1 : Inport
  Action Port : ActionPort
  Out1 : Outport
  wires:
  In1/1 -> Out1/1

== system urineanalylsis/Subsystem2/Subsystem1/Blood_Pressure_check/diastol_Elevated/If Action Subsystem11 ==
  In1 : Inport
  Action Port : ActionPort
  Out1 : Outport
  wires:
  In1/1 -> Out1/1

== system urineanalylsis/Subsystem2/Subsystem1/Blood_Pressure_check/systol_Ht1/If Action Subsystem2 ==
  In1 : Inport
  Action Port : ActionPort
  Out1 : Outport
  wires:
  In1/1 -> Out1/1

== system urineanalylsis/Subsystem2/Subsystem1/Blood_Pressure_check/systol_Ht1/If Action Subsystem3 ==
  In1 : Inport
  Action Port : ActionPort
  Out1 : Outport
  wires:
  In1/1 -> Out1/1

== system urineanalylsis/Subsystem2/Subsystem1/Blood_Pressure_check/systol_elevated/If Action Subsystem ==
  In1 : Inport
  Action Port : ActionPort
  Out1 : Outport
  wires:
  In1/1 -> Out1/1

== system urineanalylsis/Subsystem2/Subsystem1/Blood_Pressure_check/systol_elevated/If Action Subsystem1 ==
  In1 : Inport
  Action Port : ActionPort
  Out1 : Outport
  wires:
  In1/1 -> Out1/1

== system urineanalylsis/Subsystem2/Subsystem1/Blood_Pressure_check/systol_low/If Action Subsystem8 ==
  In1 : Inport
  Action Port : ActionPort
  Out1 : Outport
  wires:
  In1/1 -> Out1/1

== system urineanalylsis/Subsystem2/Subsystem1/Blood_Pressure_check/systol_low/If Action Subsystem9 ==
  In1 : Inport
  Action Port : ActionPort
  Out1 : Outport
  wires:
  In1/1 -> Out1/1

== system urineanalylsis/Subsystem2/Subsystem1/Blood_Pressure_check/systol_normal/If Action Subsystem20 ==
  In1 : Inport
  Action Port : ActionPort
  Out1 : Outport
  wires:
  In1/1 -> Out1/1
